simulink model "reverbTest"  (R2023a)
settings: Solver=VariableStepAuto  StartTime=0.0  StopTime=2.5  RelTol=1e-3
libraries: dspsnks4 x1, dspsigops x1, dspvision x1
settings Model: Creator=zacha  LastModifiedBy=zacha

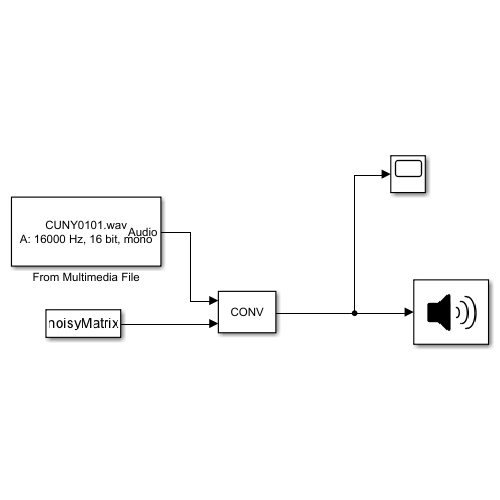
[thumbnail: Simulink's stored preview of the top-level diagram]
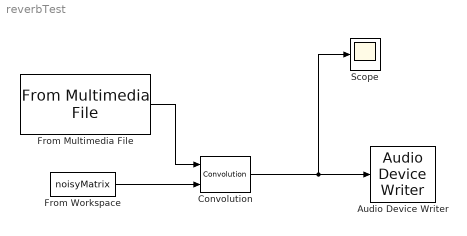
== system reverbTest ==
  Audio Device Writer : dspsnks4/Audio Device Writer  Driver=DirectSound  Device=Default  InheritSampleRate=on  SampleRate=44100  BitDepth=16-bit integer  BufferSize=4096  NumBuffers=10  DefaultOutputChannelMapping=on  OutputChannelMapping=1:2  OutputNumUnderrunSamples=off  DriverIdx=1  DeviceWarnFlag=''
  Convolution : dspsigops/Convolution  domain=Time  roundingMode=Floor  overflowMode=off  outputDataTypeStr=Inherit: Same as accumulator  outputMin=[]  outputMax=[]  outputLastDataTypeStr=Inherit: Same as accumulator
  From Workspace : FromWorkspace  VariableName=noisyMatrix  SampleTime=1/16000  OutputAfterFinalValue=Setting to zero
  From Multimedia File : dspvision/From Multimedia File  inputFilename=C:\Users\zacha\Desktop\Cochlear\Media\zach reverb audio\zach reverb audio\CUNY0101.wav  readRange=[1 Inf]  loop=on  numPlays=1  outputStreams=Audio only  videoDataType=single  audioDataType=double  inheritSampleTime=on  userDefinedSampleTime=1/30  noAudioOutput=off  isIntensityVideo=off  fourcc=RGB  colorVideoFormat=Separate color signals  outputEOF=off  dataOrg=Column-major  audioFrameSize=1  computeAudioFrameSize=off  outSamplingMode=Sample based
      settings: LibrarySourceBlock=dspsrcs4/From Multimedia File
  Scope : Scope
  wires:
  Convolution/1 -> Scope/1, Audio Device Writer/1
  From Multimedia File/1 -> Convolution/1
  From Workspace/1 -> Convolution/2
